simulink model "triggeredsub"  (Simulink 7.6)
settings: Solver=VariableStepDiscrete  StartTime=0.0  StopTime=8  MaxStep=.1  RelTol=1e-3
libraries: simulink x1
Description:
  | Triggered Subsystems
  | 
  | This demonstration shows the concept of triggered subsystems and what the
  | different trigger types are.  A triggered subsystem is executed for one time step
  | only each time the trigger port transitions from false to true in a certain direction.
  | The transition of the trigger port may occur when the direction of the transition
  | is rising, falling or both rising and falling.
  | 
  | A rising transition occurs when the trigger signal transitions from zero or below
  | to a positive value.  A falling transition occurs when the trigger signal transitions
  | from zero or above to a negative value.
  | 
  | After running the simulation, look closely at the top plot in the scope.  This shows
  | a sine wave, a waveform and the grounded value of zero.  As the waveform
  | transitions through zero, each of the subsystems is triggered appropriately.  The
  | output of each subsystem is equal to the current value of the sine wave at the time.
  | 
  | To help view exactly what is going on, you may want to turn the scope cross-hair on.
  | You can do this by double clicking on the block that says Scope Crosshair.  This will
  | enable a set of cross-hairs on the scope so that s you move your mouse you can line
  | corresponding values up across the plots.
settings Model: Creator=The MathWorks Inc.  ExtModeTrigMode=oneshot  ExtModeArmWhenConnect=off  ExtModeAutoUpdateStatusClock=off
settings DataIOCC: LimitDataPoints=off
settings OptimizationCC: BlockReduction=off  BooleanDataType=off  InlineInvariantSignals=on  InitFltsAndDblsToZero=on  BufferReusableBoundary=off
settings DebuggingCC: SaveWithParameterizedLinksMsg=none  SignalResolutionControl=TryResolveAllWithWarning  SolverPrmCheckMsg=none  MultiTaskDSMMsg=warning  MultiTaskCondExecSysMsg=none  IntegerOverflowMsg=none  BusObjectLabelMismatch=none
settings HardwareCC: TargetUnknown=on
settings RTWCC: IncludeERTFirstTime=on
settings GRTTargetCC: TargetFcnLib=ansi_tfl_tmw.mat

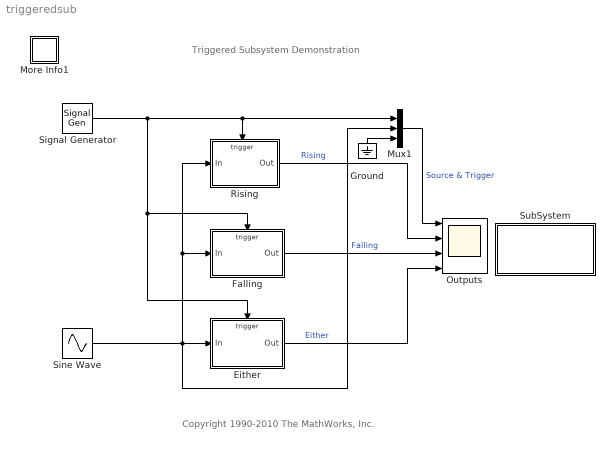
== system triggeredsub ==
  note: Triggered Subsystem Demonstration
  note: Copyright 1990-2010 The MathWorks, Inc.
  Either : Subsystem
  Falling : Subsystem
  Ground : Ground
  More Info1 : Subsystem
      settings: OpenFcn=showdemo(bdroot(gcs))
      mask Display: disp('?')
  Mux1 : Mux  Inputs=3
  Outputs : Scope  NumInputPorts=4
      settings: StartFcn=open_system(gcbh)  TickLabels=on  TimeRange=8  YMin=-1.5~-1.5~-1.5~-1.5  YMax=1.5~1.5~1.5~1.5  SaveName=trigsubdata  DataFormat=Structure
  Rising : Subsystem
  Signal Generator : SignalGenerator  WaveForm=square  Amplitude=0.5
      settings: AttributesFormatString=Waveform: %<waveform>\nFreq: %<Frequency> %<Units>
  Sine Wave : Sin  Frequency=8  SampleTime=0
      settings: AttributesFormatString=Freq: %<Frequency> rad/sec
  SubSystem : Subsystem  mask(Scope Crosshair){sch=off}
      mask prompts: sch "Scope crosshair"
      mask help: Turn on/off the crosshair pointer on the scope named Outputs.
      mask init:
      | if strcmp(get_param(gcs, 'Open'), 'off')
      |     open_system(gcs);
      | end 
      | f=get_param([gcs '/Outputs'],'Figure');
      | if strcmp(sch,'on'),
      |   ptr='fullcrosshair';
      | else,
      |   ptr= 'arrow';
      | end
      | set(f,'pointer',ptr)
      settings: OpenFcn=if strcmp(get_param(gcb,'sch'),'on'),val='off';else,val='on';end;set_param(gcb,'sch',val)
      mask Display: disp(['Scope\nCrosshair\n' sch])
  wires:
  Signal Generator/1 -> Rising/Trigger, Mux1/1, Either/Trigger, Falling/Trigger
  Sine Wave/1 -> Falling/1(In), Rising/1(In), Either/1(In), Mux1/2
  Ground/1 -> Mux1/3
  Rising/1(Out) -> Outputs/2  "Rising"
  Falling/1(Out) -> Outputs/3  "Falling"
  Either/1(Out) -> Outputs/4  "Either"
  Mux1/1 -> Outputs/1  "Source & Trigger"

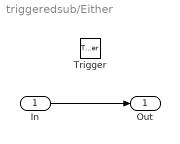
== system triggeredsub/Either ==
  In : Inport
  Trigger : TriggerPort  TriggerType=either
  Out : Outport  InitialOutput=0
  wires:
  In/1 -> Out/1

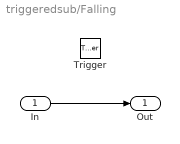
== system triggeredsub/Falling ==
  In : Inport
  Trigger : TriggerPort  TriggerType=falling
  Out : Outport  InitialOutput=0
  wires:
  In/1 -> Out/1

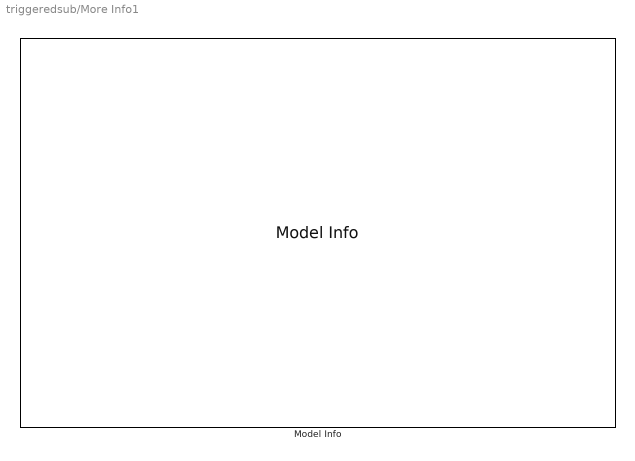
== system triggeredsub/More Info1 ==
  Model Info : simulink/Model-Wide Utilities/Model Info  SystemSampleTime=-1  InitialBlockCM=none  BlockCM=none  Frame=on  HorizontalTextAlignment=Left  LeftAlignmentValue=0.02  SourceBlockDiagram=triggeredsub  TagMaxNumber=20

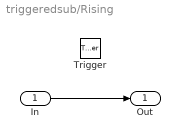
== system triggeredsub/Rising ==
  In : Inport
  Trigger : TriggerPort
  Out : Outport  InitialOutput=0
  wires:
  In/1 -> Out/1

== system triggeredsub/SubSystem ==
